simulink model "math_filter"  (Simulink 6.0)
settings: Solver=ode45  StartTime=0.0  StopTime=10.0  RelTol=1e-3
undefined symbols (not defined in the file or in its folder): Fs
libraries: rfmathmodels1 x2, dspsnks4 x1, simulink x1, dspsrcs4 x1
settings Model: Creator=ashivapr  LastModifiedBy=cvora  ProdHWDeviceType=Specified
settings DataIOCC: SaveOutput=off  SaveTime=off  SignalLoggingName=logsOut
settings DebuggingCC: CheckExecutionContextPreStartOutputMsg=on  CheckExecutionContextRuntimeOutputMsg=on  SolverPrmCheckMsg=none
settings HardwareCC: ProdHWDeviceType=Specified
settings ModelReferenceCC: UpdateModelReferenceTargets=IfOutOfDate
settings CodeAppCC: MangleLength=5
settings GRTTargetCC: LifeSpan=inf
settings SFSimCC: SFSimApplyToAllLibs=on  SFSimBuildMode=Incremental

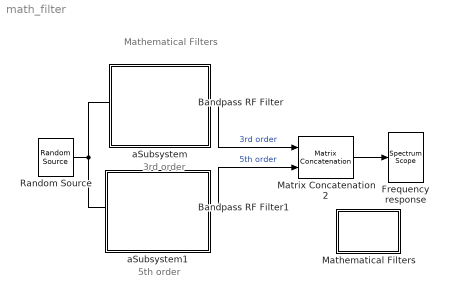
== system math_filter ==
  note: Mathematical Filters
  note: 5th order
  note: 3rd order
  Bandpass RF Filter : rfmathmodels1/Bandpass RF Filter  method=Chebyshev I  filttype=Bandpass  N=3  flo=72e6  fhi=78e6  Rp=1  Rs=10  MaxLength=32  Fc=75e6  Ts=1e-7
  Bandpass RF Filter1 : rfmathmodels1/Bandpass RF Filter  method=Chebyshev I  filttype=Bandpass  N=5  flo=72e6  fhi=78e6  Rp=1  Rs=10  MaxLength=32  Fc=75e6  Ts=1e-7
  Frequency response : dspsnks4/Spectrum Scope  ScopeProperties=off  Domain=Frequency  HorizSpan=1  UseBuffer=off  BufferSize=128  Overlap=64  inpFftLenInherit=off  FFTlength=1024  numAvg=400  DisplayProperties=off  AxisGrid=on  Memory=off  FrameNumber=off  AxisLegend=on  AxisZoom=off  OpenScopeAtSimStart=on  OpenScopeImmediately=off  FigPos=[5 328 704 266]  AxisProperties=on  XUnits=Hertz  XRange=[-Fs/2...Fs/2]  InheritXIncr=on  XIncr=1.0  XLabel=Samples  YUnits=dB  YLabel=Magnitude, dB  LineProperties=off  LineColors=[0 0 1]|[1 0 0]
      settings: YMin=-6  YMax=1
  Mathematical Filters : Subsystem  EnableExecutionContextPropagation=on
      mask Display: disp('Info')
  Matrix Concatenation2 : simulink/Math Operations/Matrix Concatenation  numInports=2  catMethod=Horizontal
  Random Source : dspsrcs4/Random Source  SrcType=Gaussian  NormMethod=Ziggurat  CltLength=12  Min=0  Max=1  Mean=0  Var=1  RepMode=Not repeatable  Seed=1  Inherit=off  SampMode=Discrete  SampTime=1e-7  SampFrame=256  DataType=Double  OutComplex=Complex
  aSubsystem : Subsystem  EnableExecutionContextPropagation=on
      mask Display: disp('')
  aSubsystem1 : Subsystem  EnableExecutionContextPropagation=on
      mask Display: disp('')
  wires:
  Random Source/1 -> Bandpass RF Filter/1, Bandpass RF Filter1/1
  Matrix Concatenation2/1 -> Frequency response/1
  Bandpass RF Filter1/1 -> Matrix Concatenation2/2  "5th order"
  Bandpass RF Filter/1 -> Matrix Concatenation2/1  "3rd order"

== system math_filter/Mathematical Filters ==
  note: Mathematical Filters
  note: This model compares two Chebyshev I filters of order 3 and 5
      | with a passband ripple of 1dB implemented using
      | Bandpass RF filters from the Mathematical sub-library.
  note: Filter specifications:
      | Center frequency = 75MHz
      | Lower passband edge frequency = 72MHz
      | Upper passband edge frequency  = 78MHz
      | Hence, bandwidth of the filter at -1dB = (78-72) =6MHz
  note: The frequency response of the 5th order filter has five ripples and
      | the frequency response of the 3rd order filter has three ripples
      | as expected. Also, observe that the roll-off of the 5th order filter
      | is steeper compared to the roll-off of the 3rd order filter.

== system math_filter/aSubsystem ==

== system math_filter/aSubsystem1 ==
